simulink model "Plane_animation"  (R2016a)
settings: Solver=FixedStepDiscrete  StartTime=0.0  StopTime=10000  FixedStep=.1  RelTol=1e-3
undefined symbols (not defined in the file or in its folder): drawPlane
libraries: simulink x6
settings Model: Creator=beard  LastModifiedBy=waffles
settings DataIOCC: LimitDataPoints=on  SaveFormat=Array  SignalLoggingSaveFormat=ModelDataLogs
settings OptimizationCC: ExpressionDepthLimit=2147483647  InitFltsAndDblsToZero=on
settings DebuggingCC: UnderspecifiedInitializationDetection=Classic  MergeDetectMultiDrivingBlocksExec=none  SolverPrmCheckMsg=warning  FcnCallInpInsideContextMsg=UseLocalSettings  StateNameClashWarn=warning
settings HardwareCC: ProdBitPerPointer=32  ProdLargestAtomicFloat=None  ProdIntDivRoundTo=Undefined  ProdEndianess=Unspecified  ProdWordSize=32  ProdHWDeviceType=32-bit Generic
settings ModelReferenceCC: PropagateSignalLabelsOutOfModel=off
settings GRTTargetCC: CombineOutputUpdateFcns=off  GRTInterface=on
settings ConfigComp: CovModelRefEnable=Off  CovSFcnEnable=off

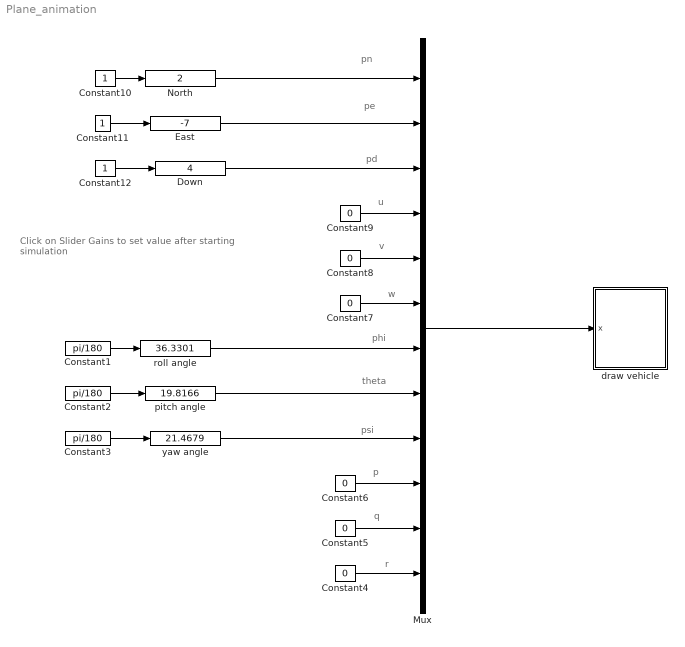
== system Plane_animation ==
  note: pn
  note: pe
  note: pd
  note: phi
  note: theta
  note: psi
  note: p
  note: q
  note: r
  note: u
  note: v
  note: w
  note: Click on Slider Gains to set value
      | after starting simulation
  Constant1 : Constant  Value=pi/180
  Constant10 : Constant
  Constant11 : Constant
  Constant12 : Constant
  Constant2 : Constant  Value=pi/180
  Constant3 : Constant  Value=pi/180
  Constant{4..9} (6 alike) : Constant  Value=0
  Down : simulink/Math Operations/Slider Gain  low=-10  gain=4  high=10
  East : simulink/Math Operations/Slider Gain  low=-10  gain=-7  high=10
  Mux : Mux  Inputs=12
  North : simulink/Math Operations/Slider Gain  low=-10  gain=2  high=10
  draw vehicle : Subsystem
      mask Display: image(imread('tv.jpg'))
  pitch angle : simulink/Math Operations/Slider Gain  low=-180  gain=19.8166  high=180
  roll angle : simulink/Math Operations/Slider Gain  low=-180  gain=36.3301  high=180
  "yaw angle " : simulink/Math Operations/Slider Gain  low=-180  gain=21.4679  high=180
  wires:
  Mux/1 -> draw vehicle/1(x)
  roll angle/1 -> Mux/7
  Constant1/1 -> roll angle/1
  pitch angle/1 -> Mux/8
  Constant2/1 -> pitch angle/1
  "yaw angle "/1 -> Mux/9
  Constant3/1 -> "yaw angle "/1
  Constant4/1 -> Mux/12
  Constant5/1 -> Mux/11
  Constant6/1 -> Mux/10
  Constant7/1 -> Mux/6
  Constant8/1 -> Mux/5
  Constant9/1 -> Mux/4
  North/1 -> Mux/1
  Constant10/1 -> North/1
  East/1 -> Mux/2
  Constant11/1 -> East/1
  Down/1 -> Mux/3
  Constant12/1 -> Down/1

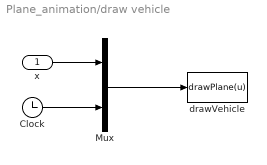
== system Plane_animation/draw vehicle ==
  x : Inport
  Clock : Clock
  Mux : Mux  Inputs=2
  drawVehicle : MATLABFcn  MATLABFcn=drawPlane(u)  OutputDimensions=0  SampleTime=0.1
  wires:
  Mux/1 -> drawVehicle/1
  x/1 -> Mux/1
  Clock/1 -> Mux/2
